simulink model "simulacao"  (R2024a)
settings: Solver=VariableStepAuto  StartTime=0.0  StopTime=34e-3  RelTol=1e-3
libraries: eeTransforms x1, spsabctodq0Lib x1
settings Model: Creator=lcce-  LastModifiedBy=lcce-

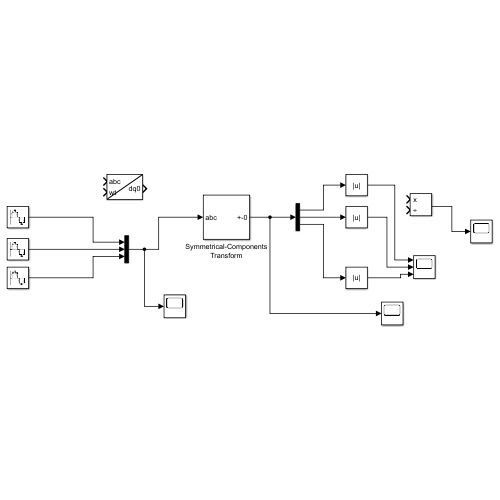
[thumbnail: Simulink's stored preview of the top-level diagram]
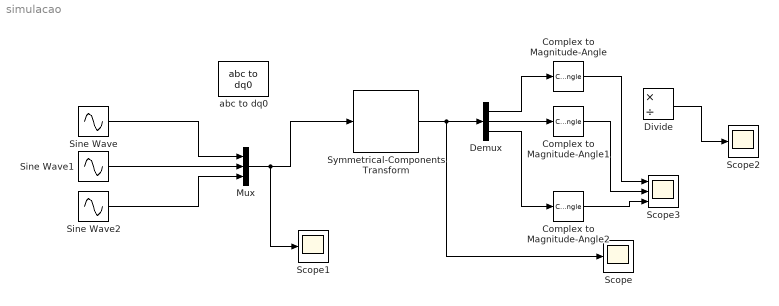
== system simulacao ==
  Complex to Magnitude-Angle : ComplexToMagnitudeAngle  Output=Magnitude
  Complex to Magnitude-Angle1 : ComplexToMagnitudeAngle  Output=Magnitude
  Complex to Magnitude-Angle2 : ComplexToMagnitudeAngle  Output=Magnitude
  Demux : Demux  Outputs=3
  Divide : Product  Inputs=*/
  Mux : Mux  Inputs=3
  Scope : Scope
  Scope1 : Scope
  Scope2 : Scope
  Scope3 : Scope  NumInputPorts=3
  Sine Wave : Sin  Amplitude=sqrt(2)/sqrt(3) * 220  Frequency=2*pi*60  SampleTime=1/9000
  Sine Wave1 : Sin  Amplitude=sqrt(2)/sqrt(3) * 220 * 0.5  Frequency=2*pi*60  Phase=2*pi/3  SampleTime=1/9000
  Sine Wave2 : Sin  Amplitude=sqrt(2)/sqrt(3) * 220  Frequency=2*pi*60  Phase=-2*pi/3  SampleTime=1/9000
  Symmetrical-Components Transform : eeTransforms/Symmetrical-Components Transform  PowerInvariant=off
      settings: LibrarySourceBlock=|
      | ee_sl_lib/Mathematical
      | Transforms/Symmetrical-Components
      | Transform
  abc to dq0 : spsabctodq0Lib/abc to dq0  Alignment=90 degrees behind phase A axis
  wires:
  Symmetrical-Components Transform/1 -> Scope/1, Demux/1
  Sine Wave/1 -> Mux/1
  Sine Wave1/1 -> Mux/2
  Sine Wave2/1 -> Mux/3
  Mux/1 -> Scope1/1, Symmetrical-Components Transform/1
  Divide/1 -> Scope2/1
  Demux/2 -> Complex to Magnitude-Angle1/1
  Demux/1 -> Complex to Magnitude-Angle/1
  Demux/3 -> Complex to Magnitude-Angle2/1
  Complex to Magnitude-Angle/1 -> Scope3/1
  Complex to Magnitude-Angle1/1 -> Scope3/2
  Complex to Magnitude-Angle2/1 -> Scope3/3
